simulink model "MPC"  (R2021a)
settings: Solver=VariableStepAuto  StartTime=0.0  StopTime=10.0  RelTol=1e-3
values from neighbouring files (symbols this model uses):
  Bg = 1    [Run_Ship_PI.m]
  Bs = mean(B)    [Run_Ship_PI.m]
  Cg = 1    [Run_Ship_PI.m]
  Cs = abs(mean(C))    [Run_Ship_PI.m]
  Ig = 1    [Run_Ship_PI.m]
  Is = ((1/12)*2)+(0.5+0.6^2)    (= 1.02666666667)    [Run_Ship_PI.m]
  Kd = 600    [Run_Ship_PI.m]
  Kg = Wspin*Ispin    (= 1)    [Run_Ship_PI.m]
  Kp = 30    [Run_Ship_PI.m]
  w = 1    [Run_Ship_PI.m]
libraries: simulink x1, mpclib x1
settings Model: Creator=samcl  LastModifiedBy=samcl

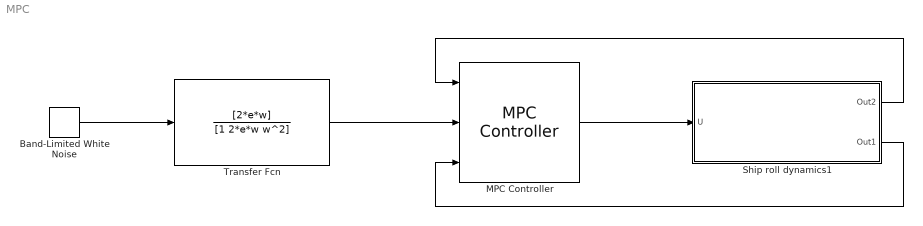
== system MPC ==
  Band-Limited White Noise : simulink/Sources/Band-Limited White Noise  Cov=[0.1]  Ts=0.1  seed=[23341]
  MPC Controller : mpclib/MPC Controller  SCDEnableBlockLinearizationSpecification=on  is_multiple=0  enable_value=0  return_u0=off  updateMPCinCallerWorkspace=on  md_inport=on  mv_inport=off  uref_inport=off  return_cost=off  return_mvseq=off  return_qpstatus=off  return_xseq=off  return_state=off  return_ovseq=off  state_inport=off  umin_inport=off  umax_inport=off  ymin_inport=off  ymax_inport=off  cc_inport=off  ywt_inport=off  uwt_inport=off  duwt_inport=off  rhoeps_inport=off  pm_inport=off  MaximumP=10  HorizonChoice=FixedHorizon  n_ts=1  n_p=10  n_mv=1  n_md=0  n_ud=0  n_mo=1  n_uo=0  BlockDataType=double  SampleTimeInherited=off  switch_inport=off
  Ship roll dynamics1 : Subsystem  Description=plant
      settings: MinAlgLoopOccurrences=on
  Transfer Fcn : TransferFcn  Numerator=[2*e*w]  Denominator=[1 2*e*w w^2]
  wires:
  Ship roll dynamics1/1(Out2) -> MPC Controller/1
  MPC Controller/1 -> Ship roll dynamics1/1(U)
  Transfer Fcn/1 -> MPC Controller/2
  Ship roll dynamics1/2(Out1) -> MPC Controller/3
  Band-Limited White Noise/1 -> Transfer Fcn/1

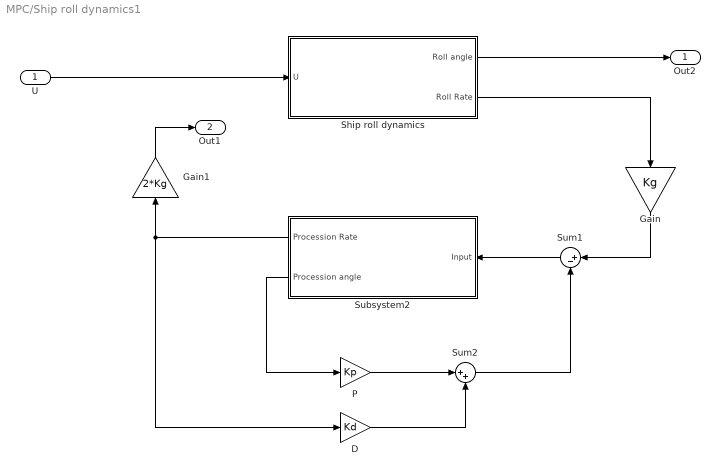
== system MPC/Ship roll dynamics1 ==
  U : Inport
  D : Gain  Gain=Kd
  Gain : Gain  Gain=Kg
  Gain1 : Gain  Gain=2*Kg
  P : Gain  Gain=Kp
  Ship roll dynamics : Subsystem  Description=plant
      settings: MinAlgLoopOccurrences=on
  Subsystem2 : Subsystem
  Sum1 : Sum  Inputs=|+-
  Sum2 : Sum  Inputs=|++
  Out2 : Outport
  Out1 : Outport  Port=2
  wires:
  Ship roll dynamics/1(Roll angle) -> Out2/1
  Ship roll dynamics/2(Roll Rate) -> Gain/1
  Gain/1 -> Sum1/1
  Subsystem2/1(Procession Rate) -> Gain1/1, D/1
  U/1 -> Ship roll dynamics/1(U)
  D/1 -> Sum2/2
  Sum2/1 -> Sum1/2
  Sum1/1 -> Subsystem2/1(Input)
  Subsystem2/2(Procession angle) -> P/1
  P/1 -> Sum2/1
  Gain1/1 -> Out1/1

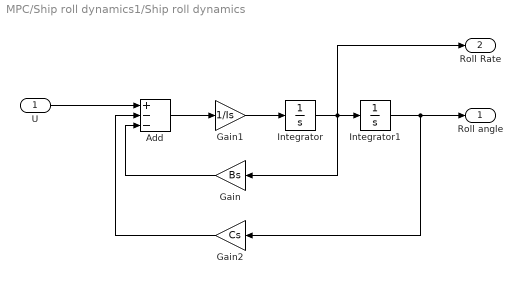
== system MPC/Ship roll dynamics1/Ship roll dynamics ==
  U : Inport
  Add : Sum  Inputs=+--
  Gain : Gain  Gain=Bs
  Gain1 : Gain  Gain=1/Is
  Gain2 : Gain  Gain=Cs
  Integrator : Integrator
  Integrator1 : Integrator
  Roll angle : Outport
  Roll Rate : Outport  Port=2
  wires:
  U/1 -> Add/1
  Add/1 -> Gain1/1
  Gain1/1 -> Integrator/1
  Integrator/1 -> Gain/1, Roll Rate/1, Integrator1/1
  Integrator1/1 -> Gain2/1, Roll angle/1
  Gain2/1 -> Add/2
  Gain/1 -> Add/3

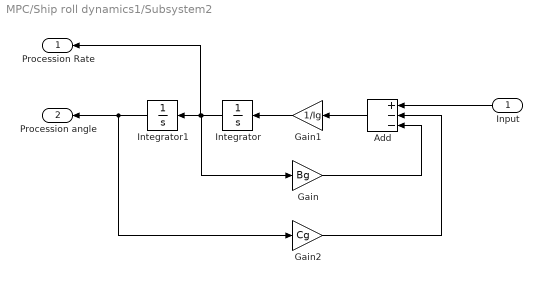
== system MPC/Ship roll dynamics1/Subsystem2 ==
  Input : Inport
  Add : Sum  Inputs=+--
  Gain : Gain  Gain=Bg
  Gain1 : Gain  Gain=1/Ig
  Gain2 : Gain  Gain=Cg
  Integrator : Integrator
  Integrator1 : Integrator
  Procession Rate : Outport
  Procession angle : Outport  Port=2
  wires:
  Input/1 -> Add/1
  Add/1 -> Gain1/1
  Integrator1/1 -> Procession angle/1, Gain2/1
  Gain/1 -> Add/3
  Gain2/1 -> Add/2
  Integrator/1 -> Procession Rate/1, Integrator1/1, Gain/1
  Gain1/1 -> Integrator/1
